simulink model "FOCSalvatore"  (R2022a)
settings: Solver=VariableStepAuto  StartTime=0.0  StopTime=10.0  RelTol=1e-3
values from neighbouring files (symbols this model uses):
  p = 6    [Data.m]    (also in FOC_BANG_Script.m; IFOCdatav6.m)
  Tr = Lm*(1+sigma_r)/Rr    [FOC_BANG_Script.m]    (also in IFOCdatav6.m)
  Vdc = 350    [Data.m]    (also in FOC_BANG_Script.m; IFOCdatav6.m)
undefined symbols (not defined in the file or in its folder): deltae
libraries: spsControlledVoltageSourceLib x3, spsCurrentMeasurementLib x3, slpidlib x1, spsAsynchronousMachineSIUnitsLib x1, spspowerguiLib x1
settings Model: Creator=salvatoregranata  LastModifiedBy=salvatoregranata

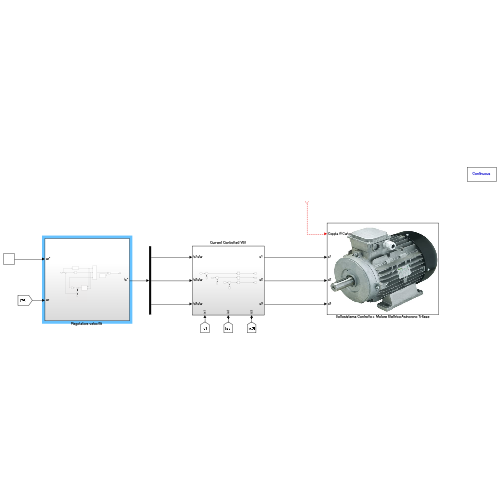
[thumbnail: Simulink's stored preview of the top-level diagram]
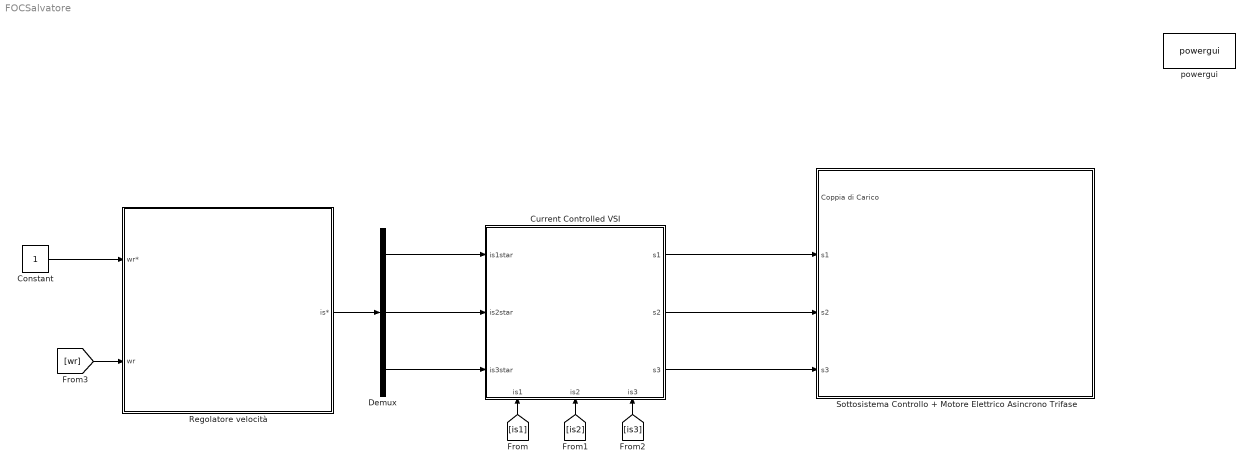
== system FOCSalvatore ==
  Constant : Constant
  Current Controlled VSI : Subsystem
      settings: PortSchema="{\"entries\":[{\"content\":{\"sides\":[{\"content\":{\"connectorIds\":[\"In1\",\"In2\",\"In3\"]},\"type\":\"ConnectorPlacement.EquallySpacedRectSide\",\"uuid\":\"70c47f39-1d77-41dd-a694-32b88b6bee6a\"},{\"content\":{\"connectorIds\":[\"Out1\",\"Out2\",\"Out3\"],\"side\":\"RIGHT\"},\"type\":\"ConnectorPlacement.EquallySpacedRectSide\",\"uuid\":\"1bbe43ef-9979-4657-8bf3-bf813a7552bf\"},{\"content\":{\"connectorIds\":[],\"side\":\"TOP\"},\"type\":\"ConnectorPlacement.EquallySpacedRectSide\",\"uuid\":\"4134b8e5-8067-4738-bdb7-1e562e3cc3f9\"},{\"content\":{\"connectorIds\":[\"In4\",\"In5\",\"In6\"],\"side\":\"BOTTOM\"},\"type\":\"ConnectorPlacement.EquallySpacedRectSide\",\"uuid\":\"34c08927-af3a-4329-864a-5e141f406158\"}]},\"type\":\"ConnectorPlacement.EquallySpacedConnector\",\"uuid\":\"b4b4ed0b-775c-4454-8acf-d68ddb9bca3b\"}],\"packageUris\":[\"http://schema.mathworks.com/mf0/Connector/R2020b\"],\"version\":\"1.0\"}"
  Demux : Demux  Outputs=3
  "Regolatore velocità " : Subsystem
  Sottosistema Controllo + Motore Elettrico Asincrono Trifase : Subsystem
      mask Display: image('/Users/salvatoregranata/Downloads/Asincroni_Trifa11.jpg'); % Use "Edit Image" on toolstrip to change.
  powergui : spspowerguiLib/powergui  Priority=1  SimulationMode=Continuous  SampleTime=50e-6  frequency=60  Iterations=50  frequencyindice=60  Pbase=100e6  ErrMax=1e-4  UnitsV=kV  UnitsW=MW  buscounter=0  FunctionMessages=off  echomessages=off  EnableUseOfTLC=off  CurrentSourceSwitches=off  DisableSnubberDevices=off  DisableRonSwitches=off  DisableVfSwitches=off  DisplayEquations=off  AutomaticDiscreteSolvers=off  SolverType=Tustin/Backward Euler (TBE)  Interpol=off  ExternalGateDelay=off  methode=off  Ts=100  x0status=blocks  SPID=on  SwTol=0  HookPort=off  NonlinearTolerance=1e-4  nMaxIteration=100  ContinueOnMaxIteration=off  RestoreLinks=warning  ResistiveCurrentMeasurement=off  Frange=[0:2:500]  Ylog=off  Xlog=on  ShowGrid=off  save=off  variable=ZData  structure=0  ZoomFFT=off  StartTime=0.0  cycles=1  DisplayStyle=1  fundamental=60  FreqAxis=off  MaxFrequency=1000  frequencyindicesteady=1  RmsSteady=1  display=off
  wires:
  Current Controlled VSI/1(s1) -> Sottosistema Controllo + Motore Elettrico Asincrono Trifase/2(s1)
  Current Controlled VSI/2(s2) -> Sottosistema Controllo + Motore Elettrico Asincrono Trifase/3(s2)
  Current Controlled VSI/3(s3) -> Sottosistema Controllo + Motore Elettrico Asincrono Trifase/4(s3)
  [is1] -> Current Controlled VSI/4(is1)
  [is3] -> Current Controlled VSI/6(is3)
  [is2] -> Current Controlled VSI/5(is2)
  [wr] -> "Regolatore velocità "/2(wr)
  "Regolatore velocità "/1(is*) -> Demux/1
  Demux/2 -> Current Controlled VSI/2(is2star)
  Demux/1 -> Current Controlled VSI/1(is1star)
  Demux/3 -> Current Controlled VSI/3(is3star)
  ? -> Sottosistema Controllo + Motore Elettrico Asincrono Trifase/1(Coppia di Carico)
  Constant/1 -> "Regolatore velocità "/1(wr*)

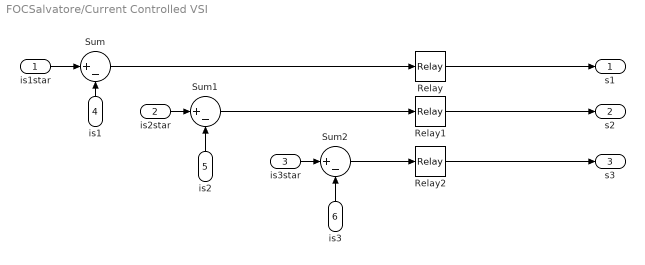
== system FOCSalvatore/Current Controlled VSI ==
  is1star : Inport
  is2star : Inport  Port=2
  is3star : Inport  Port=3
  is1 : Inport  Port=4
  is2 : Inport  Port=5
  is3 : Inport  Port=6
  Relay : Relay  OnSwitchValue=deltae  OffSwitchValue=-deltae
  Relay1 : Relay  OnSwitchValue=deltae  OffSwitchValue=-deltae
  Relay2 : Relay  OnSwitchValue=deltae  OffSwitchValue=-deltae
  Sum : Sum  Inputs=|+-
  Sum1 : Sum  Inputs=|+-
  Sum2 : Sum  Inputs=|+-
  s1 : Outport
  s2 : Outport  Port=2
  s3 : Outport  Port=3
  wires:
  Relay1/1 -> s2/1
  Relay/1 -> s1/1
  Relay2/1 -> s3/1
  Sum1/1 -> Relay1/1
  Sum/1 -> Relay/1
  Sum2/1 -> Relay2/1
  is1star/1 -> Sum/1
  is3star/1 -> Sum2/1
  is2star/1 -> Sum1/1
  is2/1 -> Sum1/2
  is1/1 -> Sum/2
  is3/1 -> Sum2/2

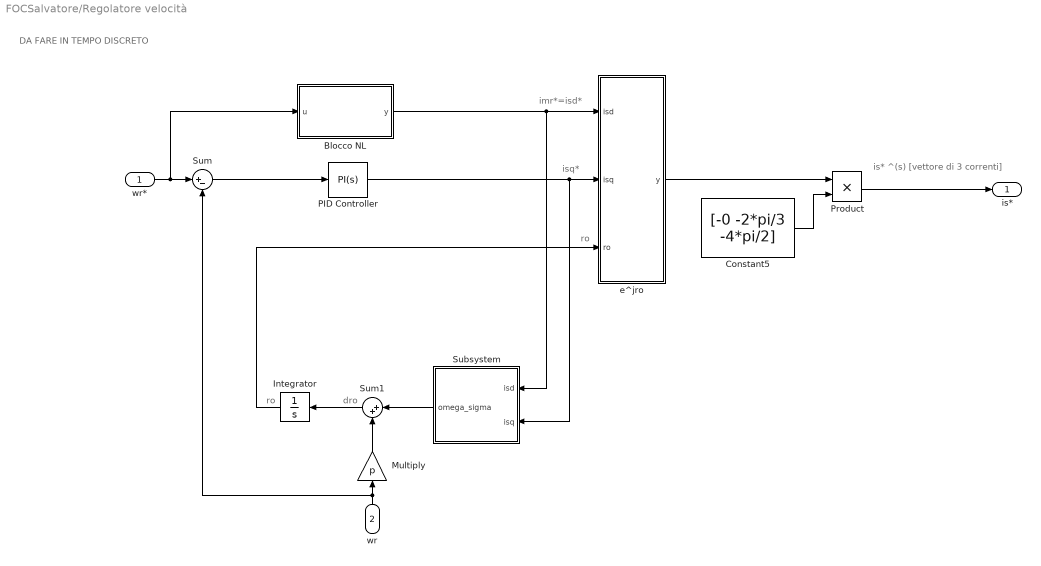
== system FOCSalvatore/Regolatore velocità  ==
  note: is* ^(s) [vettore di 3 correnti]
  note: DA FARE IN TEMPO DISCRETO
  note: ro
  note: isq*
  note: imr*=isd*
  note: ro
  note: dro
  wr* : Inport
  wr : Inport  Port=2
  Blocco NL : MATLAB Function  TreatAsAtomicUnit=on
  Constant5 : Constant  Value=[-0 -2*pi/3 -4*pi/2]
  Integrator : Integrator
  Multiply : Gain  Gain=p
  PID Controller : slpidlib/PID Controller  Controller=PI  Form=Parallel  TimeDomain=Continuous-time  UseExternalTs=off  SampleTime=-1  IntegratorMethod=Forward Euler  FilterMethod=Forward Euler  ControllerParametersSource=internal  P=1  I=1  UseKiTs=off  D=0  N=100  UseFilter=on  TunerSelectOption=Transfer Function Based (PID Tuner App)  InitialConditionSource=internal  InitialConditionForIntegrator=0  InitialConditionForFilter=0  DifferentiatorICPrevScaledInput=0  ExternalReset=none  TrackingMode=off  Kt=1  LimitOutput=off  SatLimitsSource=internal  UpperSaturationLimit=inf  LowerSaturationLimit=-inf  LinearizeAsGain=on  AntiWindupMode=none  Kb=1  POutMin=[]  POutMax=[]  IOutMin=[]  IOutMax=[]  DOutMin=[]  DOutMax=[]  NOutMin=[]  NOutMax=[]  SumOutMin=[]  SumOutMax=[]  SaturationOutMin=[]  SaturationOutMax=[]  PParamMin=[]  PParamMax=[]  IParamMin=[]  IParamMax=[]  DParamMin=[]  DParamMax=[]  NParamMin=[]  NParamMax=[]  KbParamMin=[]  KbParamMax=[]  KtParamMin=[]  KtParamMax=[]  KbOutMin=[]  KbOutMax=[]  KtOutMin=[]  KtOutMax=[]  IntegratorOutMin=[]  IntegratorOutMax=[]  FilterOutMin=[]  FilterOutMax=[]  SumI1OutMin=[]  SumI1OutMax=[]  SumI2OutMin=[]  SumI2OutMax=[]  SumI3OutMin=[]  SumI3OutMax=[]  SumI4OutMin=[]  SumI4OutMax=[]  SumDOutMin=[]  SumDOutMax=[]  DifferentiatorOutMin=[]  DifferentiatorOutMax=[]  FilterDiffOutCoefMin=[]  FilterDiffOutCoefMax=[]  ReciprocalOutMin=[]  ReciprocalOutMax=[]  SumDenOutMin=[]  SumDenOutMax=[]  SumNumOutMin=[]  SumNumOutMax=[]  DivideOutMin=[]  DivideOutMax=[]  UdiffTsProdOutMin=[]  UdiffTsProdOutMax=[]  NTsProdOutMin=[]  NTsProdOutMax=[]  UintegralTsProdOutMin=[]  UintegralTsProdOutMax=[]  UngainTsProdOutMin=[]  UngainTsProdOutMax=[]  IntegratorContinuousStateAttributes=''  IntegratorStateMustResolveToSignalObject=off  IntegratorRTWStateStorageClass=Auto  FilterContinuousStateAttributes=''  FilterStateMustResolveToSignalObject=off  FilterRTWStateStorageClass=Auto  ParallelPVariant=InternalParameters  IdealPVariant=Disabled  IVariant=InternalParameters  DVariant=Disabled  IntegratorVariant=Continuous  SatVariant=Disabled  AWVariant=Passthrough  PCopyVariant=Disabled  TRVariant=Disabled  FdbkBlocksVariant=Forward  IdealPFdbkVariant=Disabled  SatFdbkVariant=Disabled  DerivativeFilterVariant=Disabled  NVariant=Disabled  NCopyVariant=Disabled_SignalSpec  FilterICVariant=Disabled  IntegratorICVariant=InternalICs  ExternalResetVariant=Disabled  TRSumVariant=Passthrough  SumFdbkVariant=Disabled  SumVariant=Sum_PI  TsampFilterVariant=InternalTs  TsampNgainVariant=Passthrough  TsampIntegralVariant=Passthrough  ExternalSaturationOutDataTypeStr=Inherit: Same as second input  aMode=0
  Product : Product
  Subsystem : Subsystem
  Sum : Sum  Inputs=|+-
  Sum1 : Sum  Inputs=|++
  e^jro : MATLAB Function  TreatAsAtomicUnit=on
  is* : Outport
  wires:
  Sum/1 -> PID Controller/1
  PID Controller/1 -> e^jro/2(isq), Subsystem/2(isq)
  Blocco NL/1(y) -> Subsystem/1(isd), e^jro/1(isd)
  Integrator/1 -> e^jro/3(ro)
  Subsystem/1(omega_sigma) -> Sum1/1
  Multiply/1 -> Sum1/2
  wr/1 -> Sum/2, Multiply/1
  Sum1/1 -> Integrator/1
  wr*/1 -> Blocco NL/1(u), Sum/1
  e^jro/1(y) -> Product/1
  Constant5/1 -> Product/2
  Product/1 -> is*/1

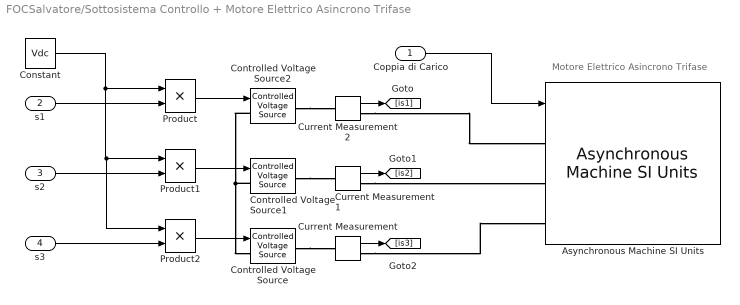
== system FOCSalvatore/Sottosistema Controllo + Motore Elettrico Asincrono Trifase ==
  note: Motore Elettrico Asincrono Trifase
  Coppia di Carico : Inport
  s1 : Inport  Port=2
  s2 : Inport  Port=3
  s3 : Inport  Port=4
  Asynchronous Machine SI Units : spsAsynchronousMachineSIUnitsLib/Asynchronous Machine SI Units  RotorType=Squirrel-cage  PresetModel=No  MechanicalLoad=Torque Tm  ShowDetailedParameters=on  ReferenceFrame=Rotor  Units=SI  MeasurementBus=off  NominalParameters=[1.845e+04 400 50]  VoltageRatio=1  Stator=[0.5968 0.0003495]  Rotor=[0.6258 0.005473]  Cage1=[0.4155 0.002066]  Cage2=[0.4168 0.0003495]  Lm=0.0354  Mechanical=[0.05 0.005879 2]  PolePairs=2  InitialConditions=[0 0 0 0 0 0 0 0]  SimulateSaturation=off  Saturation=[14.03593122, 27.81365428, 53.79336849, 72.68890987, 97.98006896, 148.6815601, 215.7428561, 302.9841135, 428.7778367 ; 230, 322, 414, 460, 506, 552, 598, 644, 690]  LoadFlowParameters=1492000  TsPowergui=0  TsBlock=-1  IterativeModel=Trapezoidal non iterative  IterativeDiscreteModel=Trapezoidal non iterative  Pmec=1.492e+006
  Constant : Constant  Value=Vdc
  Controlled Voltage Source : spsControlledVoltageSourceLib/Controlled Voltage Source  Initialize=on  Source_Type=AC  Amplitude=0  Phase=0  Frequency=0  Measurements=None
  Controlled Voltage Source1 : spsControlledVoltageSourceLib/Controlled Voltage Source  Initialize=on  Source_Type=AC  Amplitude=0  Phase=0  Frequency=0  Measurements=None
  Controlled Voltage Source2 : spsControlledVoltageSourceLib/Controlled Voltage Source  Initialize=on  Source_Type=AC  Amplitude=0  Phase=0  Frequency=0  Measurements=None
  Current Measurement : spsCurrentMeasurementLib/Current Measurement  PhasorSimulation=off  OutputType=Complex  PSBequivalent=0
  Current Measurement1 : spsCurrentMeasurementLib/Current Measurement  PhasorSimulation=off  OutputType=Complex  PSBequivalent=0
  Current Measurement2 : spsCurrentMeasurementLib/Current Measurement  PhasorSimulation=off  OutputType=Complex  PSBequivalent=0
  Product : Product
  Product1 : Product
  Product2 : Product
  wires:
  Coppia di Carico/1 -> Asynchronous Machine SI Units/1
  Constant/1 -> Product2/1, Product1/1, Product/1
  Product/1 -> Controlled Voltage Source2/1
  Product1/1 -> Controlled Voltage Source1/1
  Product2/1 -> Controlled Voltage Source/1
  s1/1 -> Product/2
  s2/1 -> Product1/2
  s3/1 -> Product2/2
  Current Measurement2/1 -> [is1]
  Current Measurement/1 -> [is3]
  Current Measurement1/1 -> [is2]
  connections:
  Controlled Voltage Source/RConn1 -- Current Measurement/LConn1
  Current Measurement/RConn1 -- Asynchronous Machine SI Units/LConn3
  Controlled Voltage Source2/RConn1 -- Current Measurement2/LConn1
  Current Measurement2/RConn1 -- Asynchronous Machine SI Units/LConn1
  Controlled Voltage Source1/RConn1 -- Current Measurement1/LConn1
  Current Measurement1/RConn1 -- Asynchronous Machine SI Units/LConn2
  Controlled Voltage Source2/LConn1 -- Controlled Voltage Source1/LConn1 -- Controlled Voltage Source/LConn1

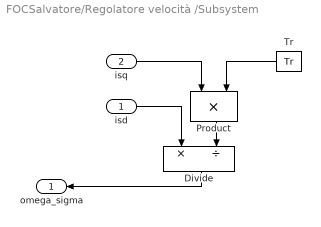
== system FOCSalvatore/Regolatore velocità /Subsystem ==
  isd : Inport
  isq : Inport  Port=2
  Divide : Product  Inputs=*/
  Product : Product
  Tr : Constant  Value=Tr
  omega_sigma : Outport
  wires:
  isd/1 -> Divide/1
  Divide/1 -> omega_sigma/1
  Tr/1 -> Product/2
  isq/1 -> Product/1
  Product/1 -> Divide/2

== matlab function FOCSalvatore/Regolatore velocità /Blocco NL ==
  data: u input; y output
function y = fcn(u)

y = u;

== matlab function FOCSalvatore/Regolatore velocità /e^jro ==
  data: isd input; y output; isq input; ro input
function y = fcn(isd,isq,ro)
